simulink model "twozonevav"  (R2020a)
settings: Solver=FixedStepAuto  StartTime=0.0  StopTime=Inf  FixedStep=0.001  RelTol=1e-3
PostLoadFcn:
  | if any(exist('dsrtsu_mdlpostloadfcn', 'file') ~= 0), dsrtsu_mdlpostloadfcn('Execute', bdroot); end
InitFcn:
  | , if any(exist('rtifpga_mdlclblib', 'file') ~= 0), rtifpga_mdlclblib('Init', bdroot); end,
  | , if any(exist('dsmpb_private', 'file') ~= 0), dsmpb_private('dsmpb_mdlclblib', 'Init', bdroot); end,
libraries: dsmpblib x8
(part 3 of 3)

== system twozonevav/behavior/dymola/Dymola Settings ==

== system twozonevav/behavior/dymola/Modelica model2 ==

== system twozonevav/behavior/dymola/compmodel ==

== system twozonevav/behavior/dymola/editmodel ==
